simulink model "models"  (R2022b)
settings: Solver=VariableStepAuto  StartTime=0.0  StopTime=2  RelTol=1e-3
settings Model: Creator=jack  LastModifiedBy=jack

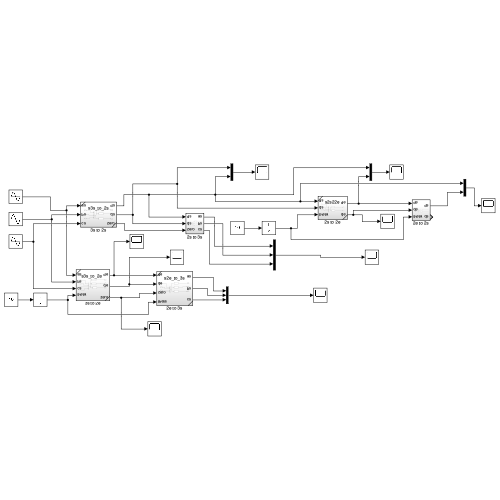
[thumbnail: Simulink's stored preview of the top-level diagram]
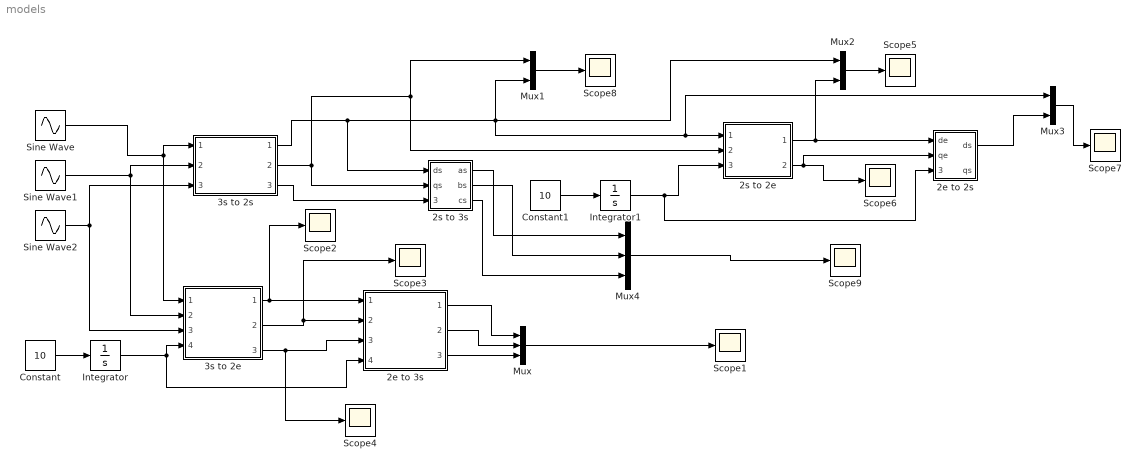
== system models ==
  2e to 2s : Subsystem
  2e to 3s : Subsystem  ReferencedSubsystem=s2e_to_3s
  2s to 2e : Subsystem  ReferencedSubsystem=s2s22e
  2s to 3s : Subsystem
  3s to 2e : Subsystem  ReferencedSubsystem=s3s_to_2e
  3s to 2s : Subsystem  ReferencedSubsystem=s3s_to_2s
  Constant : Constant  Value=10
  Constant1 : Constant  Value=10
  Integrator : Integrator
  Integrator1 : Integrator
  Mux : Mux  Inputs=3
  Mux1 : Mux  Inputs=2
  Mux2 : Mux  Inputs=2
  Mux3 : Mux  Inputs=2
  Mux4 : Mux  Inputs=3
  Scope{1..9} (9 alike) : Scope
  Sine Wave : Sin  Frequency=10
  Sine Wave1 : Sin  Frequency=10  Phase=-2*pi/3
  Sine Wave2 : Sin  Frequency=10  Phase=2*pi/3
  wires:
  Sine Wave/1 -> 3s to 2e/1, 3s to 2s/1
  Sine Wave2/1 -> 3s to 2e/3, 3s to 2s/3
  3s to 2s/1 -> 2s to 3s/1(ds), Mux2/1, Mux1/2, Mux3/1, 2s to 2e/1
  3s to 2s/2 -> 2s to 3s/2(qs), Mux1/1, 2s to 2e/2
  Constant/1 -> Integrator/1
  3s to 2e/1 -> Scope2/1, 2e to 3s/1
  3s to 2e/3 -> Scope4/1, 2e to 3s/3
  Mux/1 -> Scope1/1
  2e to 3s/1 -> Mux/1
  2e to 3s/2 -> Mux/2
  2e to 3s/3 -> Mux/3
  3s to 2e/2 -> Scope3/1, 2e to 3s/2
  2s to 2e/2 -> 2e to 2s/2(qe), Scope6/1
  Integrator/1 -> 2e to 3s/4, 3s to 2e/4
  Mux1/1 -> Scope8/1
  Mux2/1 -> Scope5/1
  2s to 2e/1 -> 2e to 2s/1(de), Mux2/2
  Constant1/1 -> Integrator1/1
  Integrator1/1 -> 2e to 2s/3(theta), 2s to 2e/3
  Sine Wave1/1 -> 3s to 2s/2, 3s to 2e/2
  2e to 2s/1(ds) -> Mux3/2
  Mux3/1 -> Scope7/1
  3s to 2s/3 -> 2s to 3s/3(zero)
  2s to 3s/1(as) -> Mux4/1
  2s to 3s/2(bs) -> Mux4/2
  2s to 3s/3(cs) -> Mux4/3
  Mux4/1 -> Scope9/1

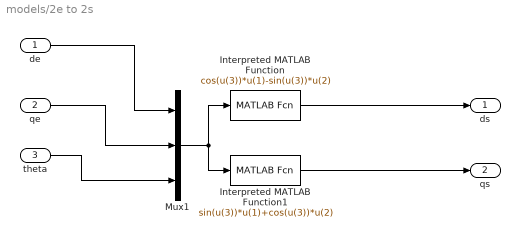
== system models/2e to 2s ==
  de : Inport
  qe : Inport  Port=2
  theta : Inport  Port=3
  Interpreted MATLAB Function : MATLABFcn  MATLABFcn=cos(u(3))*u(1)-sin(u(3))*u(2)
  Interpreted MATLAB Function1 : MATLABFcn  MATLABFcn=sin(u(3))*u(1)+cos(u(3))*u(2)
  Mux1 : Mux  Inputs=3
  ds : Outport
  qs : Outport  Port=2
  wires:
  theta/1 -> Mux1/3
  Interpreted MATLAB Function/1 -> ds/1
  qe/1 -> Mux1/2
  de/1 -> Mux1/1
  Interpreted MATLAB Function1/1 -> qs/1
  Mux1/1 -> Interpreted MATLAB Function/1, Interpreted MATLAB Function1/1

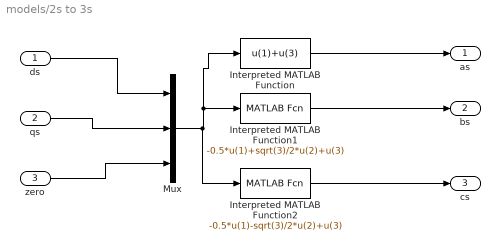
== system models/2s to 3s ==
  ds : Inport
  qs : Inport  Port=2
  zero : Inport  Port=3
  Interpreted MATLAB Function : MATLABFcn  MATLABFcn=u(1)+u(3)
  Interpreted MATLAB Function1 : MATLABFcn  MATLABFcn=-0.5*u(1)+sqrt(3)/2*u(2)+u(3)
  Interpreted MATLAB Function2 : MATLABFcn  MATLABFcn=-0.5*u(1)-sqrt(3)/2*u(2)+u(3)
  Mux : Mux  Inputs=3
  as : Outport
  bs : Outport  Port=2
  cs : Outport  Port=3
  wires:
  qs/1 -> Mux/2
  ds/1 -> Mux/1
  Mux/1 -> Interpreted MATLAB Function1/1, Interpreted MATLAB Function/1, Interpreted MATLAB Function2/1
  zero/1 -> Mux/3
  Interpreted MATLAB Function2/1 -> cs/1
  Interpreted MATLAB Function/1 -> as/1
  Interpreted MATLAB Function1/1 -> bs/1
